simulink model "HPC_service"  (R2024a)
settings: Solver=FixedStepDiscrete  StartTime=0.0  StopTime=10.0  RelTol=1e-3
undefined symbols (not defined in the file): orig
settings Model: Creator=diell  LastModifiedBy=diell

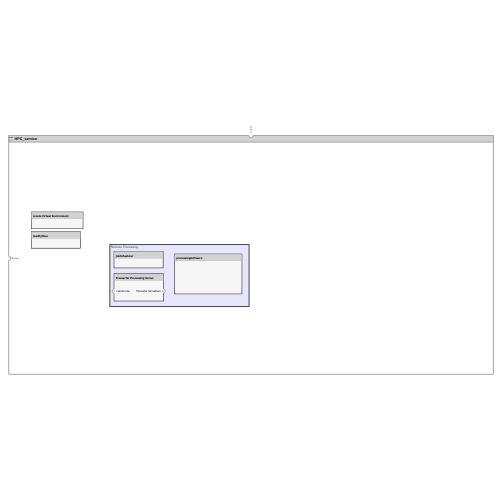
[thumbnail: Simulink's stored preview of the top-level diagram]
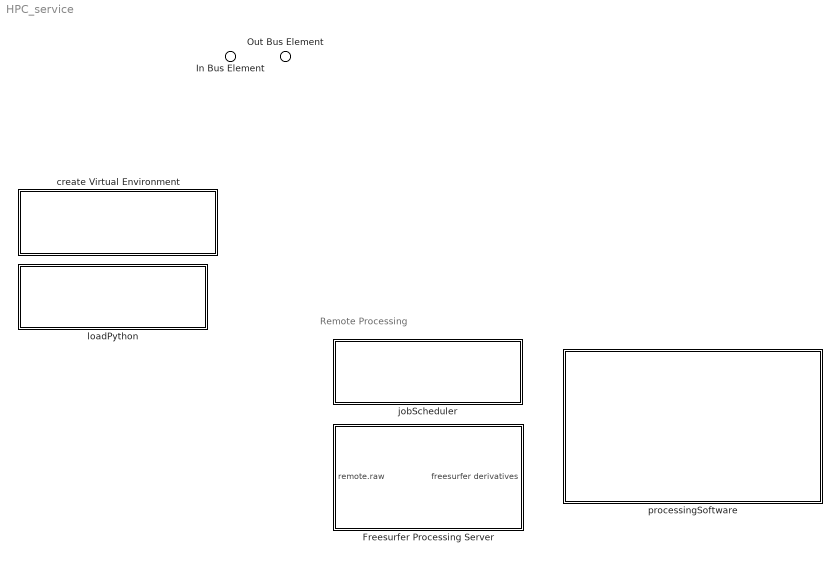
== system HPC_service ==
  note: Remote Processing
  In Bus Element : Inport  AllowServiceAccess=on  PortName=Client
  Freesurfer Processing Server : Subsystem
      settings: PortSchema="{\"entries\":[{\"content\":{\"headerSize\":26,\"margin\":15,\"minimumSpacing\":25,\"sides\":[{\"content\":{\"connectorIds\":[\"In1\"]},\"type\":\"ConnectorPlacement.EquallySpacedRectSide\",\"uuid\":\"d99db108-8c8a-4010-81b2-f142fbf318f5\"},{\"content\":{\"connectorIds\":[\"Out1\"],\"side\":\"RIGHT\"},\"type\":\"ConnectorPlacement.EquallySpacedRectSide\",\"uuid\":\"9190d96c-22e3-4cc9-a507-8f094dc67743\"},{\"content\":{\"side\":\"TOP\"},\"type\":\"ConnectorPlacement.EquallySpacedRectSide\",\"uuid\":\"08b46875-eac1-4edb-b2eb-5598dd517a75\"},{\"content\":{\"side\":\"BOTTOM\"},\"type\":\"ConnectorPlacement.EquallySpacedRectSide\",\"uuid\":\"ace7fe11-fb05-49db-a7ee-0fa9beffa30a\"}]},\"type\":\"ConnectorPlacement.EquallySpacedConnector\",\"uuid\":\"c8d2d02b-cf5a-431f-8876-22d36c8a9b33\"}],\"packageUris\":[\"http://schema.mathworks.com/mf0/Connector/R2020b\"],\"version\":\"1.0\"}"
  create Virtual Environment : Subsystem
      settings: PortSchema="{\"entries\":[{\"content\":{\"headerSize\":26,\"margin\":15,\"minimumSpacing\":25,\"sides\":[{\"content\":{},\"type\":\"ConnectorPlacement.EquallySpacedRectSide\",\"uuid\":\"a3539b9a-22db-4da3-b271-35b287ced3a1\"},{\"content\":{\"side\":\"RIGHT\"},\"type\":\"ConnectorPlacement.EquallySpacedRectSide\",\"uuid\":\"72d9f298-5062-46d4-b3c5-f2fa85d7a7a6\"},{\"content\":{\"side\":\"TOP\"},\"type\":\"ConnectorPlacement.EquallySpacedRectSide\",\"uuid\":\"050469fd-3881-4b53-a813-94df038aa659\"}]},\"type\":\"ConnectorPlacement.EquallySpacedConnector\",\"uuid\":\"6db04dad-62f3-4987-a6a9-d236db4fe2a3\"}],\"packageUris\":[\"http://schema.mathworks.com/mf0/Connector/R2020b\"],\"version\":\"1.0\"}"
  jobScheduler : Subsystem
      settings: PortSchema="{\"entries\":[{\"content\":{\"headerSize\":26,\"margin\":15,\"minimumSpacing\":25,\"sides\":[{\"content\":{},\"type\":\"ConnectorPlacement.EquallySpacedRectSide\",\"uuid\":\"a3539b9a-22db-4da3-b271-35b287ced3a1\"},{\"content\":{\"side\":\"RIGHT\"},\"type\":\"ConnectorPlacement.EquallySpacedRectSide\",\"uuid\":\"72d9f298-5062-46d4-b3c5-f2fa85d7a7a6\"},{\"content\":{\"side\":\"TOP\"},\"type\":\"ConnectorPlacement.EquallySpacedRectSide\",\"uuid\":\"050469fd-3881-4b53-a813-94df038aa659\"}]},\"type\":\"ConnectorPlacement.EquallySpacedConnector\",\"uuid\":\"6db04dad-62f3-4987-a6a9-d236db4fe2a3\"}],\"packageUris\":[\"http://schema.mathworks.com/mf0/Connector/R2020b\"],\"version\":\"1.0\"}"
  loadPython : Subsystem
      settings: PortSchema="{\"entries\":[{\"content\":{\"headerSize\":26,\"margin\":15,\"minimumSpacing\":25,\"sides\":[{\"content\":{},\"type\":\"ConnectorPlacement.EquallySpacedRectSide\",\"uuid\":\"a3539b9a-22db-4da3-b271-35b287ced3a1\"},{\"content\":{\"side\":\"RIGHT\"},\"type\":\"ConnectorPlacement.EquallySpacedRectSide\",\"uuid\":\"72d9f298-5062-46d4-b3c5-f2fa85d7a7a6\"},{\"content\":{\"side\":\"TOP\"},\"type\":\"ConnectorPlacement.EquallySpacedRectSide\",\"uuid\":\"050469fd-3881-4b53-a813-94df038aa659\"}]},\"type\":\"ConnectorPlacement.EquallySpacedConnector\",\"uuid\":\"6db04dad-62f3-4987-a6a9-d236db4fe2a3\"}],\"packageUris\":[\"http://schema.mathworks.com/mf0/Connector/R2020b\"],\"version\":\"1.0\"}"
  processingSoftware : Subsystem
      settings: PortSchema="{\"entries\":[{\"content\":{\"headerSize\":26,\"margin\":15,\"minimumSpacing\":25,\"sides\":[{\"content\":{},\"type\":\"ConnectorPlacement.EquallySpacedRectSide\",\"uuid\":\"a3539b9a-22db-4da3-b271-35b287ced3a1\"},{\"content\":{\"side\":\"RIGHT\"},\"type\":\"ConnectorPlacement.EquallySpacedRectSide\",\"uuid\":\"72d9f298-5062-46d4-b3c5-f2fa85d7a7a6\"},{\"content\":{\"side\":\"TOP\"},\"type\":\"ConnectorPlacement.EquallySpacedRectSide\",\"uuid\":\"050469fd-3881-4b53-a813-94df038aa659\"}]},\"type\":\"ConnectorPlacement.EquallySpacedConnector\",\"uuid\":\"6db04dad-62f3-4987-a6a9-d236db4fe2a3\"}],\"packageUris\":[\"http://schema.mathworks.com/mf0/Connector/R2020b\"],\"version\":\"1.0\"}"
  Out Bus Element : Outport  AllowServiceAccess=on  PortName=Server

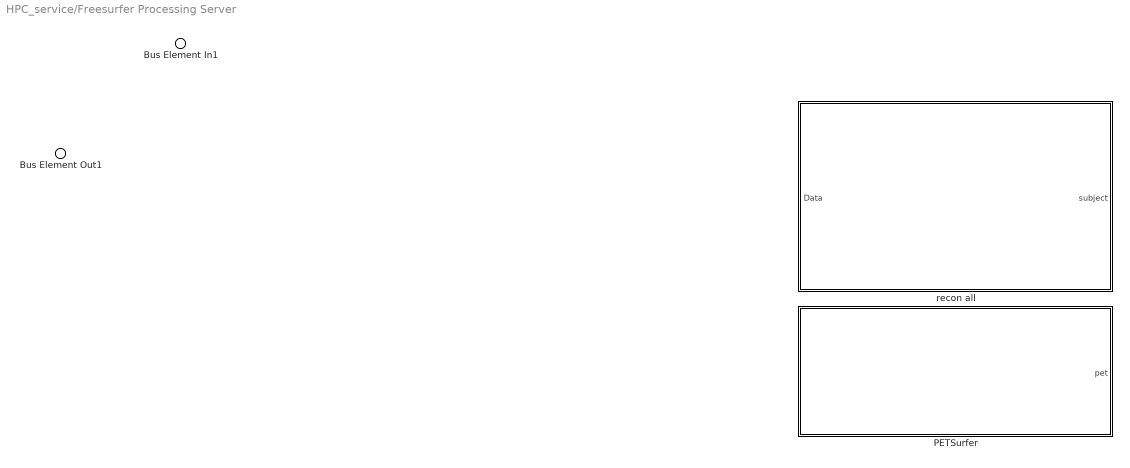
== system HPC_service/Freesurfer Processing Server ==
  Bus Element In1 : Inport  AllowServiceAccess=on  PortName=remote.raw
  PETSurfer : Subsystem
      settings: PortSchema="{\"entries\":[{\"content\":{\"headerSize\":26,\"margin\":15,\"minimumSpacing\":25,\"sides\":[{\"content\":{},\"type\":\"ConnectorPlacement.EquallySpacedRectSide\",\"uuid\":\"d99db108-8c8a-4010-81b2-f142fbf318f5\"},{\"content\":{\"connectorIds\":[\"Out1\"],\"side\":\"RIGHT\"},\"type\":\"ConnectorPlacement.EquallySpacedRectSide\",\"uuid\":\"9190d96c-22e3-4cc9-a507-8f094dc67743\"},{\"content\":{\"side\":\"TOP\"},\"type\":\"ConnectorPlacement.EquallySpacedRectSide\",\"uuid\":\"08b46875-eac1-4edb-b2eb-5598dd517a75\"}]},\"type\":\"ConnectorPlacement.EquallySpacedConnector\",\"uuid\":\"c8d2d02b-cf5a-431f-8876-22d36c8a9b33\"}],\"packageUris\":[\"http://schema.mathworks.com/mf0/Connector/R2020b\"],\"version\":\"1.0\"}"
  recon all : Subsystem
      settings: PortSchema="{\"entries\":[{\"content\":{\"headerSize\":26,\"margin\":15,\"minimumSpacing\":25,\"sides\":[{\"content\":{\"connectorIds\":[\"In1\"]},\"type\":\"ConnectorPlacement.EquallySpacedRectSide\",\"uuid\":\"1ec5f43e-86ec-4420-9dd8-c30b843d5131\"},{\"content\":{\"connectorIds\":[\"Out1\"],\"side\":\"RIGHT\"},\"type\":\"ConnectorPlacement.EquallySpacedRectSide\",\"uuid\":\"372e8174-47dc-4989-909e-f78b7a521fdc\"},{\"content\":{\"side\":\"TOP\"},\"type\":\"ConnectorPlacement.EquallySpacedRectSide\",\"uuid\":\"cc67dfee-4023-44ab-9dd9-de9f078f7d77\"}]},\"type\":\"ConnectorPlacement.EquallySpacedConnector\",\"uuid\":\"fe3e41a6-8f67-44d2-abc6-74b481cf0464\"}],\"packageUris\":[\"http://schema.mathworks.com/mf0/Connector/R2020b\"],\"version\":\"1.0\"}"
  Bus Element Out1 : Outport  PortName=freesurfer derivatives

== system HPC_service/create Virtual Environment ==

== system HPC_service/jobScheduler ==

== system HPC_service/loadPython ==

== system HPC_service/processingSoftware ==

== system HPC_service/Freesurfer Processing Server/PETSurfer ==
  Bus Element Out1 : Outport  PortName=pet

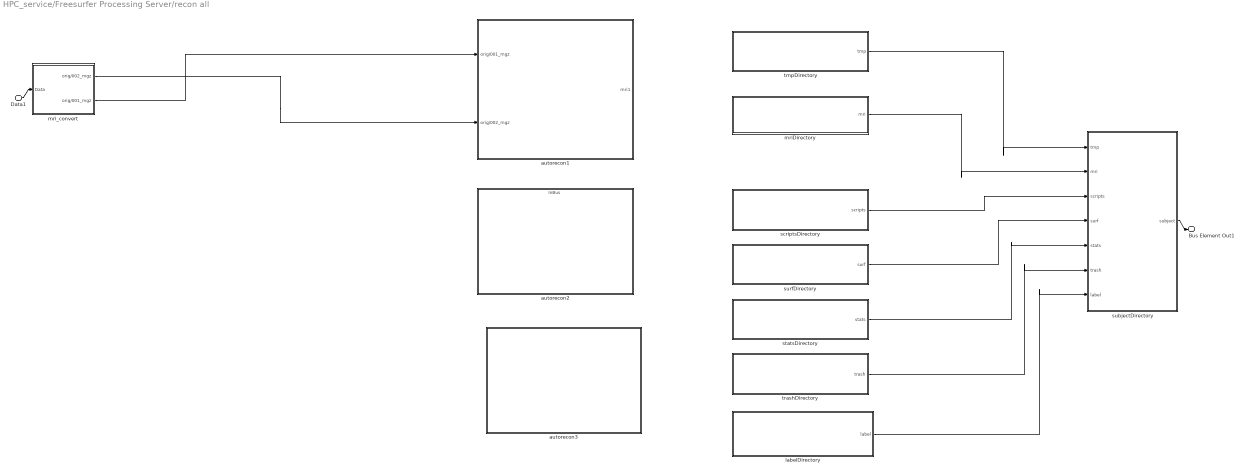
== system HPC_service/Freesurfer Processing Server/recon all ==
  Data1 : Inport  AllowServiceAccess=on  PortName=Data
  autorecon1 : Subsystem
      settings: PortSchema="{\"entries\":[{\"content\":{\"headerSize\":26,\"margin\":15,\"minimumSpacing\":25,\"sides\":[{\"content\":{\"connectorIds\":[\"In1\",\"In2\"]},\"type\":\"ConnectorPlacement.EquallySpacedRectSide\",\"uuid\":\"1ec5f43e-86ec-4420-9dd8-c30b843d5131\"},{\"content\":{\"connectorIds\":[\"Out1\"],\"side\":\"RIGHT\"},\"type\":\"ConnectorPlacement.EquallySpacedRectSide\",\"uuid\":\"372e8174-47dc-4989-909e-f78b7a521fdc\"},{\"content\":{\"side\":\"TOP\"},\"type\":\"ConnectorPlacement.EquallySpacedRectSide\",\"uuid\":\"cc67dfee-4023-44ab-9dd9-de9f078f7d77\"}]},\"type\":\"ConnectorPlacement.EquallySpacedConnector\",\"uuid\":\"fe3e41a6-8f67-44d2-abc6-74b481cf0464\"}],\"packageUris\":[\"http://schema.mathworks.com/mf0/Connector/R2020b\"],\"version\":\"1.0\"}"
  autorecon2 : Subsystem
      settings: PortSchema="{\"entries\":[{\"content\":{\"headerSize\":26,\"margin\":15,\"minimumSpacing\":25,\"sides\":[{\"content\":{},\"type\":\"ConnectorPlacement.EquallySpacedRectSide\",\"uuid\":\"d99db108-8c8a-4010-81b2-f142fbf318f5\"},{\"content\":{\"side\":\"RIGHT\"},\"type\":\"ConnectorPlacement.EquallySpacedRectSide\",\"uuid\":\"9190d96c-22e3-4cc9-a507-8f094dc67743\"},{\"content\":{\"connectorIds\":[\"In1\"],\"side\":\"TOP\"},\"type\":\"ConnectorPlacement.EquallySpacedRectSide\",\"uuid\":\"08b46875-eac1-4edb-b2eb-5598dd517a75\"}]},\"type\":\"ConnectorPlacement.EquallySpacedConnector\",\"uuid\":\"c8d2d02b-cf5a-431f-8876-22d36c8a9b33\"}],\"packageUris\":[\"http://schema.mathworks.com/mf0/Connector/R2020b\"],\"version\":\"1.0\"}"
  autorecon3 : Subsystem
      settings: PortSchema="{\"entries\":[{\"content\":{\"headerSize\":26,\"margin\":15,\"minimumSpacing\":25,\"sides\":[{\"content\":{},\"type\":\"ConnectorPlacement.EquallySpacedRectSide\",\"uuid\":\"d99db108-8c8a-4010-81b2-f142fbf318f5\"},{\"content\":{\"side\":\"RIGHT\"},\"type\":\"ConnectorPlacement.EquallySpacedRectSide\",\"uuid\":\"9190d96c-22e3-4cc9-a507-8f094dc67743\"},{\"content\":{\"side\":\"TOP\"},\"type\":\"ConnectorPlacement.EquallySpacedRectSide\",\"uuid\":\"08b46875-eac1-4edb-b2eb-5598dd517a75\"}]},\"type\":\"ConnectorPlacement.EquallySpacedConnector\",\"uuid\":\"c8d2d02b-cf5a-431f-8876-22d36c8a9b33\"}],\"packageUris\":[\"http://schema.mathworks.com/mf0/Connector/R2020b\"],\"version\":\"1.0\"}"
  labelDirectory : Subsystem
      settings: PortSchema="{\"entries\":[{\"content\":{\"headerSize\":26,\"margin\":15,\"minimumSpacing\":25,\"sides\":[{\"content\":{},\"type\":\"ConnectorPlacement.EquallySpacedRectSide\",\"uuid\":\"d99db108-8c8a-4010-81b2-f142fbf318f5\"},{\"content\":{\"connectorIds\":[\"Out1\"],\"side\":\"RIGHT\"},\"type\":\"ConnectorPlacement.EquallySpacedRectSide\",\"uuid\":\"9190d96c-22e3-4cc9-a507-8f094dc67743\"},{\"content\":{\"side\":\"TOP\"},\"type\":\"ConnectorPlacement.EquallySpacedRectSide\",\"uuid\":\"08b46875-eac1-4edb-b2eb-5598dd517a75\"}]},\"type\":\"ConnectorPlacement.EquallySpacedConnector\",\"uuid\":\"c8d2d02b-cf5a-431f-8876-22d36c8a9b33\"}],\"packageUris\":[\"http://schema.mathworks.com/mf0/Connector/R2020b\"],\"version\":\"1.0\"}"
  mriDirectory : Subsystem
      settings: PortSchema="{\"entries\":[{\"content\":{\"headerSize\":26,\"margin\":15,\"minimumSpacing\":25,\"sides\":[{\"content\":{},\"type\":\"ConnectorPlacement.EquallySpacedRectSide\",\"uuid\":\"d99db108-8c8a-4010-81b2-f142fbf318f5\"},{\"content\":{\"connectorIds\":[\"Out1\"],\"side\":\"RIGHT\"},\"type\":\"ConnectorPlacement.EquallySpacedRectSide\",\"uuid\":\"9190d96c-22e3-4cc9-a507-8f094dc67743\"},{\"content\":{\"side\":\"TOP\"},\"type\":\"ConnectorPlacement.EquallySpacedRectSide\",\"uuid\":\"08b46875-eac1-4edb-b2eb-5598dd517a75\"}]},\"type\":\"ConnectorPlacement.EquallySpacedConnector\",\"uuid\":\"c8d2d02b-cf5a-431f-8876-22d36c8a9b33\"}],\"packageUris\":[\"http://schema.mathworks.com/mf0/Connector/R2020b\"],\"version\":\"1.0\"}"
  mri_convert : Subsystem
      settings: PortSchema="{\"entries\":[{\"content\":{\"headerSize\":26,\"margin\":15,\"minimumSpacing\":25,\"sides\":[{\"content\":{\"connectorIds\":[\"In1\"]},\"type\":\"ConnectorPlacement.EquallySpacedRectSide\",\"uuid\":\"d99db108-8c8a-4010-81b2-f142fbf318f5\"},{\"content\":{\"connectorIds\":[\"Out1\",\"Out2\"],\"side\":\"RIGHT\"},\"type\":\"ConnectorPlacement.EquallySpacedRectSide\",\"uuid\":\"9190d96c-22e3-4cc9-a507-8f094dc67743\"},{\"content\":{\"side\":\"TOP\"},\"type\":\"ConnectorPlacement.EquallySpacedRectSide\",\"uuid\":\"08b46875-eac1-4edb-b2eb-5598dd517a75\"}]},\"type\":\"ConnectorPlacement.EquallySpacedConnector\",\"uuid\":\"c8d2d02b-cf5a-431f-8876-22d36c8a9b33\"}],\"packageUris\":[\"http://schema.mathworks.com/mf0/Connector/R2020b\"],\"version\":\"1.0\"}"
  scriptsDirectory : Subsystem
      settings: PortSchema="{\"entries\":[{\"content\":{\"headerSize\":26,\"margin\":15,\"minimumSpacing\":25,\"sides\":[{\"content\":{},\"type\":\"ConnectorPlacement.EquallySpacedRectSide\",\"uuid\":\"d99db108-8c8a-4010-81b2-f142fbf318f5\"},{\"content\":{\"connectorIds\":[\"Out1\"],\"side\":\"RIGHT\"},\"type\":\"ConnectorPlacement.EquallySpacedRectSide\",\"uuid\":\"9190d96c-22e3-4cc9-a507-8f094dc67743\"},{\"content\":{\"side\":\"TOP\"},\"type\":\"ConnectorPlacement.EquallySpacedRectSide\",\"uuid\":\"08b46875-eac1-4edb-b2eb-5598dd517a75\"}]},\"type\":\"ConnectorPlacement.EquallySpacedConnector\",\"uuid\":\"c8d2d02b-cf5a-431f-8876-22d36c8a9b33\"}],\"packageUris\":[\"http://schema.mathworks.com/mf0/Connector/R2020b\"],\"version\":\"1.0\"}"
  statsDirectory : Subsystem
      settings: PortSchema="{\"entries\":[{\"content\":{\"headerSize\":26,\"margin\":15,\"minimumSpacing\":25,\"sides\":[{\"content\":{},\"type\":\"ConnectorPlacement.EquallySpacedRectSide\",\"uuid\":\"d99db108-8c8a-4010-81b2-f142fbf318f5\"},{\"content\":{\"connectorIds\":[\"Out1\"],\"side\":\"RIGHT\"},\"type\":\"ConnectorPlacement.EquallySpacedRectSide\",\"uuid\":\"9190d96c-22e3-4cc9-a507-8f094dc67743\"},{\"content\":{\"side\":\"TOP\"},\"type\":\"ConnectorPlacement.EquallySpacedRectSide\",\"uuid\":\"08b46875-eac1-4edb-b2eb-5598dd517a75\"}]},\"type\":\"ConnectorPlacement.EquallySpacedConnector\",\"uuid\":\"c8d2d02b-cf5a-431f-8876-22d36c8a9b33\"}],\"packageUris\":[\"http://schema.mathworks.com/mf0/Connector/R2020b\"],\"version\":\"1.0\"}"
  subjectDirectory : Subsystem
      settings: PortSchema="{\"entries\":[{\"content\":{\"headerSize\":26,\"margin\":15,\"minimumSpacing\":25,\"sides\":[{\"content\":{\"connectorIds\":[\"In1\",\"In2\",\"In3\",\"In4\",\"In5\",\"In6\",\"In7\"]},\"type\":\"ConnectorPlacement.EquallySpacedRectSide\",\"uuid\":\"d99db108-8c8a-4010-81b2-f142fbf318f5\"},{\"content\":{\"connectorIds\":[\"Out1\"],\"side\":\"RIGHT\"},\"type\":\"ConnectorPlacement.EquallySpacedRectSide\",\"uuid\":\"9190d96c-22e3-4cc9-a507-8f094dc67743\"},{\"content\":{\"side\":\"TOP\"},\"type\":\"ConnectorPlacement.EquallySpacedRectSide\",\"uuid\":\"08b46875-eac1-4edb-b2eb-5598dd517a75\"}]},\"type\":\"ConnectorPlacement.EquallySpacedConnector\",\"uuid\":\"c8d2d02b-cf5a-431f-8876-22d36c8a9b33\"}],\"packageUris\":[\"http://schema.mathworks.com/mf0/Connector/R2020b\"],\"version\":\"1.0\"}"
  surfDirectory : Subsystem
      settings: PortSchema="{\"entries\":[{\"content\":{\"headerSize\":26,\"margin\":15,\"minimumSpacing\":25,\"sides\":[{\"content\":{},\"type\":\"ConnectorPlacement.EquallySpacedRectSide\",\"uuid\":\"d99db108-8c8a-4010-81b2-f142fbf318f5\"},{\"content\":{\"connectorIds\":[\"Out1\"],\"side\":\"RIGHT\"},\"type\":\"ConnectorPlacement.EquallySpacedRectSide\",\"uuid\":\"9190d96c-22e3-4cc9-a507-8f094dc67743\"},{\"content\":{\"side\":\"TOP\"},\"type\":\"ConnectorPlacement.EquallySpacedRectSide\",\"uuid\":\"08b46875-eac1-4edb-b2eb-5598dd517a75\"}]},\"type\":\"ConnectorPlacement.EquallySpacedConnector\",\"uuid\":\"c8d2d02b-cf5a-431f-8876-22d36c8a9b33\"}],\"packageUris\":[\"http://schema.mathworks.com/mf0/Connector/R2020b\"],\"version\":\"1.0\"}"
  tmpDirectory : Subsystem
      settings: PortSchema="{\"entries\":[{\"content\":{\"headerSize\":26,\"margin\":15,\"minimumSpacing\":25,\"sides\":[{\"content\":{},\"type\":\"ConnectorPlacement.EquallySpacedRectSide\",\"uuid\":\"d99db108-8c8a-4010-81b2-f142fbf318f5\"},{\"content\":{\"connectorIds\":[\"Out1\"],\"side\":\"RIGHT\"},\"type\":\"ConnectorPlacement.EquallySpacedRectSide\",\"uuid\":\"9190d96c-22e3-4cc9-a507-8f094dc67743\"},{\"content\":{\"side\":\"TOP\"},\"type\":\"ConnectorPlacement.EquallySpacedRectSide\",\"uuid\":\"08b46875-eac1-4edb-b2eb-5598dd517a75\"}]},\"type\":\"ConnectorPlacement.EquallySpacedConnector\",\"uuid\":\"c8d2d02b-cf5a-431f-8876-22d36c8a9b33\"}],\"packageUris\":[\"http://schema.mathworks.com/mf0/Connector/R2020b\"],\"version\":\"1.0\"}"
  trashDirectory : Subsystem
      settings: PortSchema="{\"entries\":[{\"content\":{\"headerSize\":26,\"margin\":15,\"minimumSpacing\":25,\"sides\":[{\"content\":{},\"type\":\"ConnectorPlacement.EquallySpacedRectSide\",\"uuid\":\"d99db108-8c8a-4010-81b2-f142fbf318f5\"},{\"content\":{\"connectorIds\":[\"Out1\"],\"side\":\"RIGHT\"},\"type\":\"ConnectorPlacement.EquallySpacedRectSide\",\"uuid\":\"9190d96c-22e3-4cc9-a507-8f094dc67743\"},{\"content\":{\"side\":\"TOP\"},\"type\":\"ConnectorPlacement.EquallySpacedRectSide\",\"uuid\":\"08b46875-eac1-4edb-b2eb-5598dd517a75\"}]},\"type\":\"ConnectorPlacement.EquallySpacedConnector\",\"uuid\":\"c8d2d02b-cf5a-431f-8876-22d36c8a9b33\"}],\"packageUris\":[\"http://schema.mathworks.com/mf0/Connector/R2020b\"],\"version\":\"1.0\"}"
  Bus Element Out1 : Outport  PortName=subject
  wires:
  Data1/1 -> mri_convert/1(Data)
  labelDirectory/1(label) -> subjectDirectory/7(label)
  scriptsDirectory/1(scripts) -> subjectDirectory/3(scripts)
  mriDirectory/1(mri) -> subjectDirectory/2(mri)
  trashDirectory/1(trash) -> subjectDirectory/6(trash)
  statsDirectory/1(stats) -> subjectDirectory/5(stats)
  surfDirectory/1(surf) -> subjectDirectory/4(surf)
  tmpDirectory/1(tmp) -> subjectDirectory/1(tmp)
  mri_convert/1(orig/002_mgz) -> autorecon1/2(orig/002_mgz)
  mri_convert/2(orig/001_mgz) -> autorecon1/1(orig/001_mgz)
  subjectDirectory/1(subject) -> Bus Element Out1/1

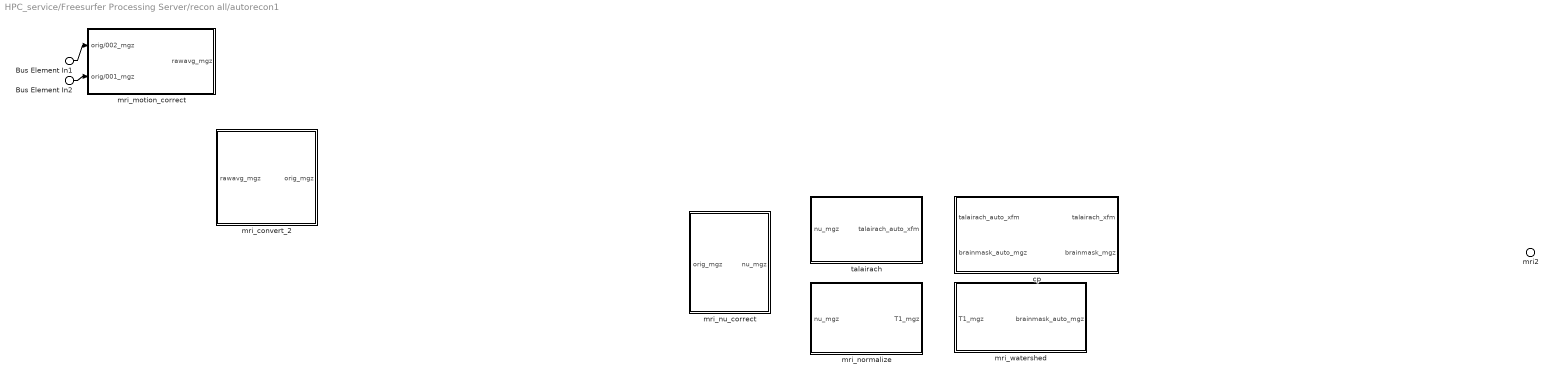
== system HPC_service/Freesurfer Processing Server/recon all/autorecon1 ==
  Bus Element In2 : Inport  PortName=orig/001_mgz
  Bus Element In1 : Inport  Port=2  PortName=orig/002_mgz
  cp : Subsystem
      settings: PortSchema="{\"entries\":[{\"content\":{\"headerSize\":26,\"margin\":15,\"minimumSpacing\":25,\"sides\":[{\"content\":{\"connectorIds\":[\"In1\",\"In2\"]},\"type\":\"ConnectorPlacement.EquallySpacedRectSide\",\"uuid\":\"d99db108-8c8a-4010-81b2-f142fbf318f5\"},{\"content\":{\"connectorIds\":[\"Out1\",\"Out2\"],\"side\":\"RIGHT\"},\"type\":\"ConnectorPlacement.EquallySpacedRectSide\",\"uuid\":\"9190d96c-22e3-4cc9-a507-8f094dc67743\"},{\"content\":{\"side\":\"TOP\"},\"type\":\"ConnectorPlacement.EquallySpacedRectSide\",\"uuid\":\"08b46875-eac1-4edb-b2eb-5598dd517a75\"}]},\"type\":\"ConnectorPlacement.EquallySpacedConnector\",\"uuid\":\"c8d2d02b-cf5a-431f-8876-22d36c8a9b33\"}],\"packageUris\":[\"http://schema.mathworks.com/mf0/Connector/R2020b\"],\"version\":\"1.0\"}"
  mri_convert_2 : Subsystem
      settings: PortSchema="{\"entries\":[{\"content\":{\"headerSize\":26,\"margin\":15,\"minimumSpacing\":25,\"sides\":[{\"content\":{\"connectorIds\":[\"In1\"]},\"type\":\"ConnectorPlacement.EquallySpacedRectSide\",\"uuid\":\"d99db108-8c8a-4010-81b2-f142fbf318f5\"},{\"content\":{\"connectorIds\":[\"Out1\"],\"side\":\"RIGHT\"},\"type\":\"ConnectorPlacement.EquallySpacedRectSide\",\"uuid\":\"9190d96c-22e3-4cc9-a507-8f094dc67743\"},{\"content\":{\"side\":\"TOP\"},\"type\":\"ConnectorPlacement.EquallySpacedRectSide\",\"uuid\":\"08b46875-eac1-4edb-b2eb-5598dd517a75\"}]},\"type\":\"ConnectorPlacement.EquallySpacedConnector\",\"uuid\":\"c8d2d02b-cf5a-431f-8876-22d36c8a9b33\"}],\"packageUris\":[\"http://schema.mathworks.com/mf0/Connector/R2020b\"],\"version\":\"1.0\"}"
  mri_motion_correct : Subsystem
      settings: PortSchema="{\"entries\":[{\"content\":{\"headerSize\":26,\"margin\":15,\"minimumSpacing\":25,\"sides\":[{\"content\":{\"connectorIds\":[\"In1\",\"In2\"]},\"type\":\"ConnectorPlacement.EquallySpacedRectSide\",\"uuid\":\"d99db108-8c8a-4010-81b2-f142fbf318f5\"},{\"content\":{\"connectorIds\":[\"Out1\"],\"side\":\"RIGHT\"},\"type\":\"ConnectorPlacement.EquallySpacedRectSide\",\"uuid\":\"9190d96c-22e3-4cc9-a507-8f094dc67743\"},{\"content\":{\"side\":\"TOP\"},\"type\":\"ConnectorPlacement.EquallySpacedRectSide\",\"uuid\":\"08b46875-eac1-4edb-b2eb-5598dd517a75\"}]},\"type\":\"ConnectorPlacement.EquallySpacedConnector\",\"uuid\":\"c8d2d02b-cf5a-431f-8876-22d36c8a9b33\"}],\"packageUris\":[\"http://schema.mathworks.com/mf0/Connector/R2020b\"],\"version\":\"1.0\"}"
  mri_normalize : Subsystem
      settings: PortSchema="{\"entries\":[{\"content\":{\"headerSize\":26,\"margin\":15,\"minimumSpacing\":25,\"sides\":[{\"content\":{\"connectorIds\":[\"In1\"]},\"type\":\"ConnectorPlacement.EquallySpacedRectSide\",\"uuid\":\"d99db108-8c8a-4010-81b2-f142fbf318f5\"},{\"content\":{\"connectorIds\":[\"Out1\"],\"side\":\"RIGHT\"},\"type\":\"ConnectorPlacement.EquallySpacedRectSide\",\"uuid\":\"9190d96c-22e3-4cc9-a507-8f094dc67743\"},{\"content\":{\"side\":\"TOP\"},\"type\":\"ConnectorPlacement.EquallySpacedRectSide\",\"uuid\":\"08b46875-eac1-4edb-b2eb-5598dd517a75\"}]},\"type\":\"ConnectorPlacement.EquallySpacedConnector\",\"uuid\":\"c8d2d02b-cf5a-431f-8876-22d36c8a9b33\"}],\"packageUris\":[\"http://schema.mathworks.com/mf0/Connector/R2020b\"],\"version\":\"1.0\"}"
  mri_nu_correct : Subsystem
      settings: PortSchema="{\"entries\":[{\"content\":{\"headerSize\":26,\"margin\":15,\"minimumSpacing\":25,\"sides\":[{\"content\":{\"connectorIds\":[\"In1\"]},\"type\":\"ConnectorPlacement.EquallySpacedRectSide\",\"uuid\":\"d99db108-8c8a-4010-81b2-f142fbf318f5\"},{\"content\":{\"connectorIds\":[\"Out1\"],\"side\":\"RIGHT\"},\"type\":\"ConnectorPlacement.EquallySpacedRectSide\",\"uuid\":\"9190d96c-22e3-4cc9-a507-8f094dc67743\"},{\"content\":{\"side\":\"TOP\"},\"type\":\"ConnectorPlacement.EquallySpacedRectSide\",\"uuid\":\"08b46875-eac1-4edb-b2eb-5598dd517a75\"}]},\"type\":\"ConnectorPlacement.EquallySpacedConnector\",\"uuid\":\"c8d2d02b-cf5a-431f-8876-22d36c8a9b33\"}],\"packageUris\":[\"http://schema.mathworks.com/mf0/Connector/R2020b\"],\"version\":\"1.0\"}"
  mri_watershed : Subsystem
      settings: PortSchema="{\"entries\":[{\"content\":{\"headerSize\":26,\"margin\":15,\"minimumSpacing\":25,\"sides\":[{\"content\":{\"connectorIds\":[\"In1\"]},\"type\":\"ConnectorPlacement.EquallySpacedRectSide\",\"uuid\":\"d99db108-8c8a-4010-81b2-f142fbf318f5\"},{\"content\":{\"connectorIds\":[\"Out1\"],\"side\":\"RIGHT\"},\"type\":\"ConnectorPlacement.EquallySpacedRectSide\",\"uuid\":\"9190d96c-22e3-4cc9-a507-8f094dc67743\"},{\"content\":{\"side\":\"TOP\"},\"type\":\"ConnectorPlacement.EquallySpacedRectSide\",\"uuid\":\"08b46875-eac1-4edb-b2eb-5598dd517a75\"}]},\"type\":\"ConnectorPlacement.EquallySpacedConnector\",\"uuid\":\"c8d2d02b-cf5a-431f-8876-22d36c8a9b33\"}],\"packageUris\":[\"http://schema.mathworks.com/mf0/Connector/R2020b\"],\"version\":\"1.0\"}"
  talairach : Subsystem
      settings: PortSchema="{\"entries\":[{\"content\":{\"headerSize\":26,\"margin\":15,\"minimumSpacing\":25,\"sides\":[{\"content\":{\"connectorIds\":[\"In1\"]},\"type\":\"ConnectorPlacement.EquallySpacedRectSide\",\"uuid\":\"d99db108-8c8a-4010-81b2-f142fbf318f5\"},{\"content\":{\"connectorIds\":[\"Out1\"],\"side\":\"RIGHT\"},\"type\":\"ConnectorPlacement.EquallySpacedRectSide\",\"uuid\":\"9190d96c-22e3-4cc9-a507-8f094dc67743\"},{\"content\":{\"side\":\"TOP\"},\"type\":\"ConnectorPlacement.EquallySpacedRectSide\",\"uuid\":\"08b46875-eac1-4edb-b2eb-5598dd517a75\"}]},\"type\":\"ConnectorPlacement.EquallySpacedConnector\",\"uuid\":\"c8d2d02b-cf5a-431f-8876-22d36c8a9b33\"}],\"packageUris\":[\"http://schema.mathworks.com/mf0/Connector/R2020b\"],\"version\":\"1.0\"}"
  mri2 : Outport  PortName=mri1
  wires:
  Bus Element In1/1 -> mri_motion_correct/1(orig/002_mgz)
  Bus Element In2/1 -> mri_motion_correct/2(orig/001_mgz)

== system HPC_service/Freesurfer Processing Server/recon all/autorecon2 ==
  Bus Element In1 : Inport  PortName=InBus

== system HPC_service/Freesurfer Processing Server/recon all/autorecon3 ==

== system HPC_service/Freesurfer Processing Server/recon all/labelDirectory ==
  Bus Element Out1 : Outport  PortName=label

== system HPC_service/Freesurfer Processing Server/recon all/mriDirectory ==
  Bus Element Out1 : Outport  PortName=mri

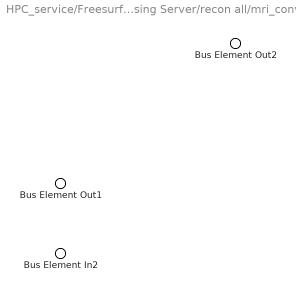
== system HPC_service/Freesurfer Processing Server/recon all/mri_convert ==
  Bus Element In2 : Inport  AllowServiceAccess=on  PortName=Data
  Bus Element Out2 : Outport  PortName=orig/002_mgz
  Bus Element Out1 : Outport  Port=2  PortName=orig/001_mgz

== system HPC_service/Freesurfer Processing Server/recon all/scriptsDirectory ==
  Bus Element Out1 : Outport  PortName=scripts

== system HPC_service/Freesurfer Processing Server/recon all/statsDirectory ==
  Bus Element Out1 : Outport  PortName=stats

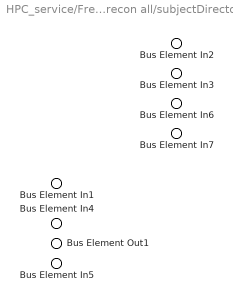
== system HPC_service/Freesurfer Processing Server/recon all/subjectDirectory ==
  Bus Element In7 : Inport  PortName=tmp
  Bus Element In6 : Inport  Port=2  PortName=mri
  Bus Element In2 : Inport  Port=3  PortName=scripts
  Bus Element In3 : Inport  Port=4  PortName=surf
  Bus Element In1 : Inport  Port=5  PortName=stats
  Bus Element In4 : Inport  Port=6  PortName=trash
  Bus Element In5 : Inport  Port=7  PortName=label
  Bus Element Out1 : Outport  PortName=subject

== system HPC_service/Freesurfer Processing Server/recon all/surfDirectory ==
  Bus Element Out1 : Outport  PortName=surf

== system HPC_service/Freesurfer Processing Server/recon all/tmpDirectory ==
  Bus Element Out1 : Outport  PortName=tmp

== system HPC_service/Freesurfer Processing Server/recon all/trashDirectory ==
  Bus Element Out1 : Outport  PortName=trash

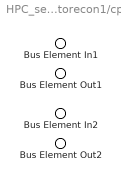
== system HPC_service/Freesurfer Processing Server/recon all/autorecon1/cp ==
  Bus Element In1 : Inport  PortName=talairach_auto_xfm
  Bus Element In2 : Inport  Port=2  PortName=brainmask_auto_mgz
  Bus Element Out1 : Outport  PortName=talairach_xfm
  Bus Element Out2 : Outport  Port=2  PortName=brainmask_mgz

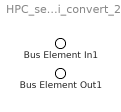
== system HPC_service/Freesurfer Processing Server/recon all/autorecon1/mri_convert_2 ==
  Bus Element In1 : Inport  PortName=rawavg_mgz
  Bus Element Out1 : Outport  PortName=orig_mgz

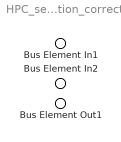
== system HPC_service/Freesurfer Processing Server/recon all/autorecon1/mri_motion_correct ==
  Bus Element In1 : Inport  PortName=orig/002_mgz
  Bus Element In2 : Inport  Port=2  PortName=orig/001_mgz
  Bus Element Out1 : Outport  PortName=rawavg_mgz

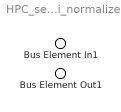
== system HPC_service/Freesurfer Processing Server/recon all/autorecon1/mri_normalize ==
  Bus Element In1 : Inport  PortName=nu_mgz
  Bus Element Out1 : Outport  PortName=T1_mgz

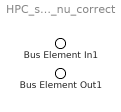
== system HPC_service/Freesurfer Processing Server/recon all/autorecon1/mri_nu_correct ==
  Bus Element In1 : Inport  PortName=orig_mgz
  Bus Element Out1 : Outport  PortName=nu_mgz

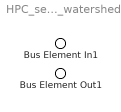
== system HPC_service/Freesurfer Processing Server/recon all/autorecon1/mri_watershed ==
  Bus Element In1 : Inport  PortName=T1_mgz
  Bus Element Out1 : Outport  PortName=brainmask_auto_mgz

== system HPC_service/Freesurfer Processing Server/recon all/autorecon1/talairach ==
  Bus Element In1 : Inport  PortName=nu_mgz
  Bus Element Out1 : Outport  PortName=talairach_auto_xfm
